simulink model "basic_sum_prod"  (R2021a)
settings: Solver=VariableStepAuto  StartTime=0.0  StopTime=10.0  RelTol=1e-3
undefined symbols (not defined in the file or in its folder): magnitude
settings Model: Creator=Aula  LastModifiedBy=Aula

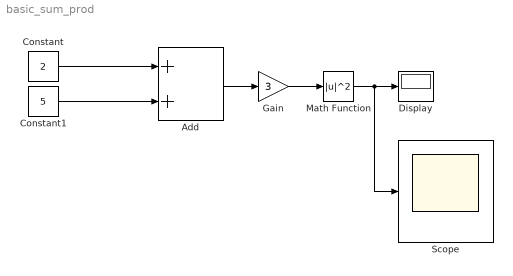
== system basic_sum_prod ==
  Add : Sum
  Constant : Constant  Value=2
  Constant1 : Constant  Value=5
  Display : Display
  Gain : Gain  Gain=3
  Math Function : Math  Operator=magnitude^2  SaturateOnIntegerOverflow=on
  Scope : Scope
  wires:
  Add/1 -> Gain/1
  Gain/1 -> Math Function/1
  Constant/1 -> Add/1
  Constant1/1 -> Add/2
  Math Function/1 -> Scope/1, Display/1
